simulink model "FYP"  (R2023b)
settings: Solver=FixedStepAuto  StartTime=0.0  StopTime=Inf  RelTol=1e-3  EnableMultiTasking=on
libraries: canmsglib x26, raspberrypiCommlib x26
(part 1 of 4)
settings Model: SimulationMode=external  ExtModeTrigDuration=2  Creator=aaron  LastModifiedBy=aaron
settings SolverCC: PositivePriorityOrder=on
settings OptimizationCC: EnhancedBackFolding=on  PassReuseOutputArgsAs=Individual arguments  ZeroExternalMemoryAtStartup=off  ZeroInternalMemoryAtStartup=off  MaxStackSize=64  OptimizeBlockOrder=speed  DifferentSizesBufferReuse=on  OptimizationCustomize=off  EfficientTunableParamExpr=on
settings DebuggingCC: UnderspecifiedInitializationDetection=Classic  MergeDetectMultiDrivingBlocksExec=none  ParameterTunabilityLossMsg=error
settings HardwareCC: ProdBitPerPointer=32  ProdBitPerSizeT=32  ProdBitPerPtrDiffT=32  ProdLargestAtomicInteger=Long  ProdLargestAtomicFloat=Double  ProdWordSize=32  ProdLongLongMode=on  ProdHWDeviceType=ARM Compatible->ARM Cortex
settings ModelReferenceCC: PropagateSignalLabelsOutOfModel=off
settings RTWCC: Description=Embedded Coder  SystemTargetFile=ert.tlc  HardwareBoard=Raspberry Pi  TemplateMakefile=ert_default_tmf  Toolchain=GNU GCC Embedded Linux  BuildConfiguration=Faster Runs
settings CodeAppCC: ForceParamTrailComments=on  IgnoreCustomStorageClasses=off  OperatorAnnotations=on  SimulinkDataObjDesc=on  SFDataObjDesc=on  InsertBlockDesc=on
settings ERTTargetCC: SupportContinuousTime=on  SupportVariableSizeSignals=on  ExtMode=on  ExtModeTransport=2  ExtModeStaticAlloc=on  ExtModeMaxTrigDuration=1000  ExtModeMexFile=ext_xcp  ExtModeMexArgs='192.168.167.94' 0 17725  ExtModeIntrfLevel=Level2 - Open

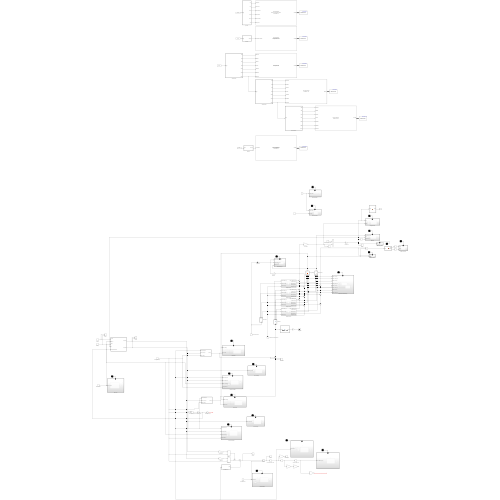
[thumbnail: Simulink's stored preview of the top-level diagram]
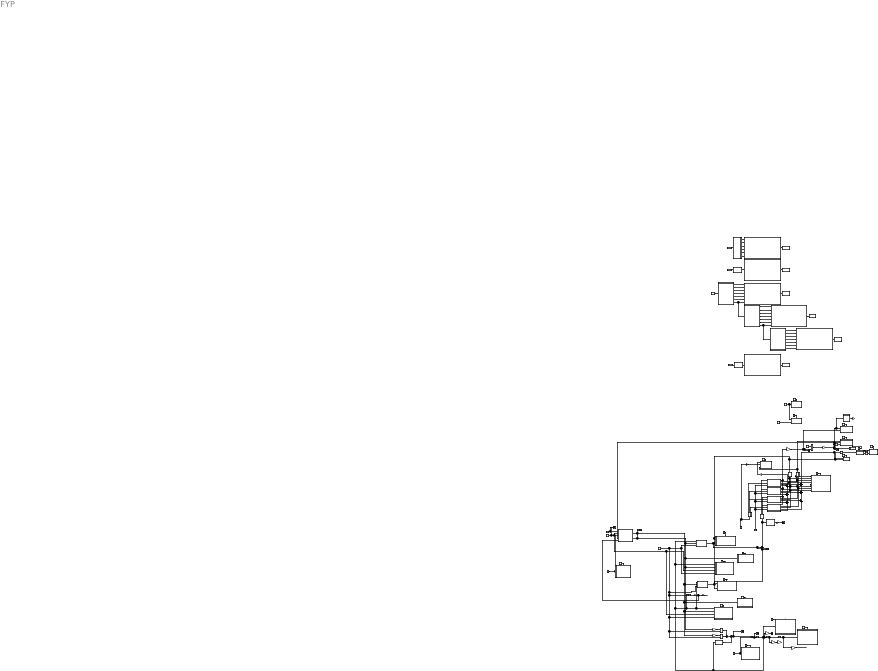
== system FYP ==
  A=F/m : Product  Inputs=*/
  Abs : Abs  SaturateOnIntegerOverflow=off
  Accel (m/s^2)to Vel (m/s) : Integrator
  Average Temp : MATLAB Function  TreatAsAtomicUnit=on
  Average Voltage : MATLAB Function  TreatAsAtomicUnit=on
  B SOC : Scope
  BMS Contactors 1 : Subsystem  TreatAsAtomicUnit=on
  BMS Contactors 2 : Subsystem  TreatAsAtomicUnit=on
  BMS Cooling Sys : Subsystem  TreatAsAtomicUnit=on
  BMS Energy Status : Subsystem  TreatAsAtomicUnit=on
  BMS Module State Monitoring : Subsystem  TreatAsAtomicUnit=on
  BMS SOC : Subsystem  TreatAsAtomicUnit=on
  BMS Sum Charge : Subsystem  TreatAsAtomicUnit=on
  BMS Sys Limits 2 : Subsystem  TreatAsAtomicUnit=on
  Battery Module 1 : Subsystem
  Battery Module 2 : Subsystem
  Battery Module 3 : Subsystem
  Battery Module 4 : Subsystem
  Brake () : Constant  Value=0
  CAN Pack1 : canmsglib/CAN Pack  MsgList=(none)  MsgName=ID405VIN  MsgIDType=Standard (11-bit identifier)  MsgIdentifier=1029  MsgLength=8  Remote=off  ApplyMinMax=off  BusOutput=on  SignalInfo={ 'VINA1405', '8', '32', 'LE', 'unsigned', 'Multiplexed', '16', '1', '0', '0', '4.29497E+009'; 'VINB405', '8', '32', 'LE', 'unsigned', 'Multiplexed', '17', '1', '0', '0', '4.29497E+009'; 'VINC405', '8', '32', 'LE', 'unsigned', 'Multiplexed', '18', '1', '0', '0', '4.29497E+009'; 'mux405', '0', '8', 'LE', 'unsigned', 'Multiplexor', '0', '1', '0', '0', '255'; 'VINA2405', '40', '24', 'LE', 'unsigned', 'Multiplexed', '16', '1', '0', '0', '1.67772E+007'; 'VINB2405', '40', '24', 'LE', 'unsigned', 'Multiplexed', '17', '1', '0', '-0', '1.67772E+007'; 'VINC2405', '40', '24', 'LE', 'unsigned', 'Multiplexed', '18', '1', '0', '0', '1.67772E+007' }
      settings: LibrarySourceBlock=canlib/CAN Pack  DataFormat=manually specified signals
  CAN Pack107 : canmsglib/CAN Pack  CANdbFile=C:\Users\aaron\OneDrive - Loughborough University\Work\Part D\FYP\tesla sniffing\Model3CAN.dbc  MsgList=ID3D8Elevation  MsgName=ID3D8Elevation  MsgIDType=Standard (11-bit identifier)  MsgIdentifier=984  MsgLength=2  Remote=off  ApplyMinMax=off  BusOutput=on  SignalInfo={'Elevation3D8','0','14','LE','signed','Standard','0','1','0','-8192','8191'}
      settings: LibrarySourceBlock=canlib/CAN Pack  DataFormat=CANdb specified signals
  CAN Pack115 : canmsglib/CAN Pack  MsgList=(none)  MsgName=ID405VIN  MsgIDType=Standard (11-bit identifier)  MsgIdentifier=1029  MsgLength=8  Remote=off  ApplyMinMax=off  BusOutput=on  SignalInfo={ 'VINA1405', '8', '32', 'LE', 'unsigned', 'Multiplexed', '16', '1', '0', '0', '4.29497E+009'; 'VINB405', '8', '32', 'LE', 'unsigned', 'Multiplexed', '17', '1', '0', '0', '4.29497E+009'; 'VINC405', '8', '32', 'LE', 'unsigned', 'Multiplexed', '18', '1', '0', '0', '4.29497E+009'; 'mux405', '0', '8', 'LE', 'unsigned', 'Multiplexor', '0', '1', '0', '0', '255'; 'VINA2405', '40', '24', 'LE', 'unsigned', 'Multiplexed', '16', '1', '0', '0', '1.67772E+007'; 'VINB2405', '40', '24', 'LE', 'unsigned', 'Multiplexed', '17', '1', '0', '-0', '1.67772E+007'; 'VINC2405', '40', '24', 'LE', 'unsigned', 'Multiplexed', '18', '1', '0', '0', '1.67772E+007' }
      settings: LibrarySourceBlock=canlib/CAN Pack  DataFormat=manually specified signals
  CAN Pack119 : canmsglib/CAN Pack  CANdbFile=C:\Users\aaron\OneDrive - Loughborough University\Work\Part D\FYP\tesla sniffing\Model3CAN.dbc  MsgList=ID528UnixTime  MsgName=ID528UnixTime  MsgIDType=Standard (11-bit identifier)  MsgIdentifier=1320  MsgLength=4  Remote=off  ApplyMinMax=off  BusOutput=on  SignalInfo={'UnixTimeSeconds528','24','32','BE','unsigned','Standard','0','1','0','0','4294970000'}
      settings: LibrarySourceBlock=canlib/CAN Pack  DataFormat=CANdb specified signals
  CAN Pack2 : canmsglib/CAN Pack  MsgList=(none)  MsgName=ID405VIN  MsgIDType=Standard (11-bit identifier)  MsgIdentifier=1029  MsgLength=8  Remote=off  ApplyMinMax=off  BusOutput=on  SignalInfo={ 'VINA1405', '8', '32', 'LE', 'unsigned', 'Multiplexed', '16', '1', '0', '0', '4.29497E+009'; 'VINB405', '8', '32', 'LE', 'unsigned', 'Multiplexed', '17', '1', '0', '0', '4.29497E+009'; 'VINC405', '8', '32', 'LE', 'unsigned', 'Multiplexed', '18', '1', '0', '0', '4.29497E+009'; 'mux405', '0', '8', 'LE', 'unsigned', 'Multiplexor', '0', '1', '0', '0', '255'; 'VINA2405', '40', '24', 'LE', 'unsigned', 'Multiplexed', '16', '1', '0', '0', '1.67772E+007'; 'VINB2405', '40', '24', 'LE', 'unsigned', 'Multiplexed', '17', '1', '0', '-0', '1.67772E+007'; 'VINC2405', '40', '24', 'LE', 'unsigned', 'Multiplexed', '18', '1', '0', '0', '1.67772E+007' }
      settings: LibrarySourceBlock=canlib/CAN Pack  DataFormat=manually specified signals
  CAN Pack82 : canmsglib/CAN Pack  CANdbFile=C:\Users\aaron\OneDrive - Loughborough University\Work\Part D\FYP\tesla sniffing\Model3CAN.dbc  MsgList=ID318SystemTimeUTC  MsgName=ID318SystemTimeUTC  MsgIDType=Standard (11-bit identifier)  MsgIdentifier=792  MsgLength=8  Remote=off  ApplyMinMax=off  BusOutput=on  SignalInfo={'UTCday318','32','8','LE','unsigned','Standard','0','1','0','-Inf','Inf';'UTChour318','24','8','LE','unsigned','Standard','0','1','0','-Inf','Inf';'UTCminutes318','40','8','LE','unsigned','Standard','0','1','0','-Inf','Inf';'UTCmonth318','8','8','LE','unsigned','Standard','0','1','0','-Inf','Inf';'UTCseconds318','16','8','LE','unsigned','Standard','0','1','0','-Inf','Inf';'UTCyear318','0','8','LE','unsigned','Standard','0','1','0','-Inf','Inf'}
      settings: LibrarySourceBlock=canlib/CAN Pack  DataFormat=CANdb specified signals
  CAN Transmit{1..2,82,107,115,119} (6 alike) : raspberrypiCommlib/CAN Transmit  DeviceID=can0  SetupCAN=off  TypeofCAN=Real  InputDataType=CAN Msg  BlockingMode_=off  BlockTimeout_=1  OutputStatus=off  IdentifierType=Standard (11-bit identifier)  MessageId=100  MsgLength=8  RemoteFrame=off  SimulateUsing=Code generation
  Coastdown Func : MATLAB Function  TreatAsAtomicUnit=on
  Constant : Constant
  Constant1 : Constant  Value=0
  Coolant Dist : MATLAB Function  TreatAsAtomicUnit=on
  Decimal to % : Gain  Gain=100
  Digital Clock1 : DigitalClock  SampleTime=1.02
  Digital Clock2 : DigitalClock
  Digital Clock3 : DigitalClock  SampleTime=1.01
  Digital Clock4 : DigitalClock
  Divide : Product  Inputs=/*
  Elevation : MATLAB Function  TreatAsAtomicUnit=on
  F=M/D front : Product  Inputs=*/
  F=M/D rear : Product  Inputs=*/
  Front PT Elec : Subsystem  TreatAsAtomicUnit=on
  Front PT Kinematics : Subsystem  TreatAsAtomicUnit=on
  Front PT Torque : Subsystem  TreatAsAtomicUnit=on
  Gain2 : Gain
  Gain3 : Gain  Gain=1/1000
  Gain5 : Gain  Gain=3.6
  Gain6 : Gain
  Gain7 : Gain  Gain=3.6
  Gain8 : Gain  Gain=3.6
  Gear Lever : Subsystem
  Gear Lever Pos : Constant  Value=3
  Integrator : Integrator
  Integrator1 : Integrator
  Integrator2 : Integrator
  M Pwr Draw : Scope  NumInputPorts=2
  MATLAB Function : MATLAB Function  TreatAsAtomicUnit=on
  MATLAB Function1 : MATLAB Function  TreatAsAtomicUnit=on
  MATLAB Function2 : MATLAB Function  TreatAsAtomicUnit=on
  MATLAB Function3 : MATLAB Function  TreatAsAtomicUnit=on
  MATLAB Function4 : MATLAB Function  TreatAsAtomicUnit=on
  MATLAB Function5 : MATLAB Function  TreatAsAtomicUnit=on
  Max Battery Capac (kWh) : Constant  Value=88
  Motor Speed (rpm) : Gain  Gain=9.54
  Motor speed (rad/s) : Gain  Gain=9.03
  Power Distr : MATLAB Function  TreatAsAtomicUnit=on
  Product : Product
  Pulse Generator{,1..18} (19 alike) : DiscretePulseGenerator  PulseType=Time based  Period=1
  Range Estimations : Subsystem  TreatAsAtomicUnit=on
  Rear PT Elec : Subsystem  TreatAsAtomicUnit=on
  Rear PT Kinematics : Subsystem  TreatAsAtomicUnit=on
  Rear PT Torque : Subsystem  TreatAsAtomicUnit=on
  Rolling Radius (m) : Constant  Value=0.3366
  Scope : Scope
  Subsystem : Subsystem
  Subsystem1 : Subsystem
  Sum{,1..9,11} (11 alike) : Sum  Inputs=++|
  Sum10 : Sum  Inputs=|+-
  Sys Time : MATLAB Function  TreatAsAtomicUnit=on
  Throttle () : Constant  Value=0
  Unix Time : MATLAB Function  TreatAsAtomicUnit=on
  V Accel : Scope
  V Force : Scope
  VIN Generation : MATLAB Function  TreatAsAtomicUnit=on
  VIN Generation1 : MATLAB Function  TreatAsAtomicUnit=on
  VIN Generation2 : MATLAB Function  TreatAsAtomicUnit=on
  Vehicle Estimates : Subsystem  TreatAsAtomicUnit=on
  Vehicle Mass )kg) : Constant  Value=1851+80*4
  Vehicle Speed : Scope
  Vel (m/s) to Disp (m) : Integrator
  W to kW : Gain  Gain=0.001
  Wh to kWh : Gain  Gain=1/1000
  assume constant flow : Constant  Value=50
  constant temp coolant from rad : Constant  Value=50
  energy perc : Scope
  gear ratio : Gain  Gain=9.03
  gear ratio1 : Gain  Gain=9.03
  kg/s to l/min : Gain  Gain=60
  pedals : Scope  NumInputPorts=2
  torques : Scope  NumInputPorts=2
  untitledPanel : Subsystem  Tag=HiddenForWebPanel  IsWebBlockPanel=on
  wheel speed (rad/s) : Product  Inputs=*/
  wires:
  Pulse Generator13/1 -> BMS Cooling Sys/Trigger
  Sum3/1 -> Wh to kWh/1
  Power Distr/2(p2) -> Battery Module 2/1(Power Request (W))
  Pulse Generator5/1 -> Front PT Kinematics/Trigger
  Sum1/1 -> Sum/2
  Pulse Generator1/1 -> Rear PT Torque/Trigger
  Pulse Generator/1 -> Rear PT Elec/Trigger
  Pulse Generator2/1 -> Rear PT Kinematics/Trigger
  Rolling Radius (m)/1 -> Rear PT Kinematics/4(Rolling Radius (m)), MATLAB Function5/3(rolling_radius_m), MATLAB Function4/3(rolling_radius_m), wheel speed (rad/s)/2, Front PT Kinematics/4(Rolling Radius (m)), F=M/D rear/2, F=M/D front/2
  Integrator/1 -> BMS SOC/3(Integrated SOC)
  Battery Module 2/4(Module Current (A)) -> Sum1/1
  Divide/1 -> Decimal to %/1
  Pulse Generator6/1 -> BMS Module State Monitoring/Trigger
  CAN Pack119/1 -> CAN Transmit119/1
  VIN Generation/1(VINA) -> CAN Pack115/1
  Sum2/1 -> Sum1/2
  Battery Module 4/3(Module Voltage (V)) -> BMS Module State Monitoring/8(Module 4 Voltage (V)), Average Voltage/4(v4)
  Battery Module 2/5(Heating Power (W)) -> Sum7/1
  Brake ()/1 -> pedals/2, Front PT Kinematics/3(Brake Pedal Pos (%)), Rear PT Kinematics/3(Brake Pedal Pos (%)), MATLAB Function1/2(brakePct)
  Product/1 -> MATLAB Function/1(power)
  MATLAB Function1/2(torqueRear) -> torques/2, Rear PT Torque/1(Motor Torque (Nm)), gear ratio1/1, Rear PT Kinematics/2(Motor Torque (m/s)), MATLAB Function5/2(motor_torque_Nm)
  Sum7/1 -> Sum8/2
  Battery Module 2/2(Module Temp (C)) -> Average Temp/2(v2), BMS Module State Monitoring/3(Module 2 Temp (C))
  MATLAB Function/1(charge) -> Integrator1/1
  CAN Pack107/1 -> CAN Transmit107/1
  Coolant Dist/3(p3) -> Battery Module 3/2(Coolant Flow (kg/s))
  Pulse Generator7/1 -> BMS Sys Limits 2/Trigger
  Integrator1/1 -> BMS Sum Charge/1(Power1)
  Integrator2/1 -> BMS Sum Charge/2(Power2)
  Pulse Generator9/1 -> BMS Energy Status/Trigger
  W to kW/1 -> BMS Cooling Sys/1(Battery Heating Power (kW))
  kg/s to l/min/1 -> BMS Cooling Sys/2(Coolant Vol Flow (LPM))
  Battery Module 3/1(Energy Remaining (Wh)) -> Sum5/1
  Battery Module 3/4(Module Current (A)) -> Sum2/1
  Pulse Generator11/1 -> BMS Contactors 2/Trigger
  Coolant Dist/2(p2) -> Battery Module 2/2(Coolant Flow (kg/s))
  Pulse Generator12/1 -> BMS Contactors 1/Trigger
  Sum6/1 -> Sum7/2
  Battery Module 4/5(Heating Power (W)) -> Sum6/2
  Battery Module 1/3(Module Voltage (V)) -> BMS Module State Monitoring/2(Module 1 Voltage (V)), Average Voltage/1(v1)
  Battery Module 3/5(Heating Power (W)) -> Sum6/1
  MATLAB Function4/1(power_W) -> Front PT Elec/2(Motor Power), M Pwr Draw/2, Sum9/2
  MATLAB Function1/1(torqueFront) -> torques/1, MATLAB Function4/2(motor_torque_Nm), Front PT Torque/1(Motor Torque (Nm)), gear ratio/1, Front PT Kinematics/2(Motor Torque (m/s))
  Max Battery Capac (kWh)/1 -> Divide/1
  Constant/1 -> BMS Contactors 2/1(Contactor State), BMS Contactors 1/1(Contactor State)
  Wh to kWh/1 -> Range Estimations/2(Energy), Scope/1, Divide/2
  CAN Pack115/1 -> CAN Transmit115/1
  Coolant Dist/1(p1) -> Battery Module 1/2(Coolant Flow (kg/s))
  Power Distr/3(p3) -> Battery Module 3/1(Power Request (W))
  Coolant Dist/4(p4) -> Battery Module 4/2(Coolant Flow (kg/s))
  Sys Time/6(year) -> CAN Pack82/6
  Battery Module 2/1(Energy Remaining (Wh)) -> Sum4/1
  Battery Module 2/3(Module Voltage (V)) -> BMS Module State Monitoring/4(Module 2 Voltage (V)), Average Voltage/2(v2)
  Average Temp/1(v) -> BMS SOC/1(Current Battery Temp), BMS Cooling Sys/3(Battery Temp (C))
  constant temp coolant from rad/1 -> Battery Module 1/3(Coolant Temp (C)), Battery Module 2/3(Coolant Temp (C)), Battery Module 3/3(Coolant Temp (C)), Battery Module 4/3(Coolant Temp (C))
  Power Distr/1(p1) -> Battery Module 1/1(Power Request (W))
  Elevation/1(Elevation) -> CAN Pack107/1
  Battery Module 4/4(Module Current (A)) -> Sum2/2
  Battery Module 3/3(Module Voltage (V)) -> BMS Module State Monitoring/6(Module 3 Voltage (V)), Average Voltage/3(v3)
  MATLAB Function/2(discharge) -> Integrator2/1
  Battery Module 3/2(Module Temp (C)) -> Average Temp/3(v3), BMS Module State Monitoring/5(Module 3 Temp (C))
  Battery Module 1/4(Module Current (A)) -> Sum/1
  Pulse Generator8/1 -> BMS Sum Charge/Trigger
  Pulse Generator3/1 -> Front PT Elec/Trigger
  MATLAB Function5/1(power_W) -> M Pwr Draw/1, Sum9/1, Rear PT Elec/2(Motor Power)
  Digital Clock3/1 -> Elevation/1(trigger)
  Accel (m/s^2)to Vel (m/s)/1 -> Coastdown Func/1(v), MATLAB Function5/1(vehicle_speed_mps), Rear PT Kinematics/1(Vehicle Speed (m/s)), wheel speed (rad/s)/1, MATLAB Function4/1(vehicle_speed_mps), Front PT Kinematics/1(Vehicle Speed (m/s)), Subsystem1/1(vehicle speed), Gain5/1, Abs/1
  Constant1/1 -> BMS Contactors 2/2(FC request)
  Battery Module 4/1(Energy Remaining (Wh)) -> Sum5/2
  Sum8/1 -> W to kW/1
  Sys Time/2(hour) -> CAN Pack82/2
  VIN Generation/2(VINB) -> CAN Pack115/2
  Battery Module 1/5(Heating Power (W)) -> Sum8/1
  Power Distr/4(p4) -> Battery Module 4/1(Power Request (W))
  CAN Pack82/1 -> CAN Transmit82/1
  Sys Time/3(minute) -> CAN Pack82/3
  Sum4/1 -> Sum3/2
  Digital Clock2/1 -> Sys Time/1(trigger)
  Sum5/1 -> Sum4/2
  Sum/1 -> BMS Sys Limits 2/1(Current), Product/1
  Unix Time/1(UnixTime) -> CAN Pack119/1
  Digital Clock1/1 -> Unix Time/1(trigger)
  Sys Time/1(day) -> CAN Pack82/1
  VIN Generation/3(VINC) -> CAN Pack115/3
  Average Voltage/1(v) -> Product/2, BMS Sys Limits 2/2(Voltage), Front PT Elec/1(Battery Voltage), Rear PT Elec/1(Battery Voltage)
  Digital Clock4/1 -> VIN Generation/1(trigger)
  Sys Time/5(second) -> CAN Pack82/5
  Pulse Generator4/1 -> Front PT Torque/Trigger
  Battery Module 1/1(Energy Remaining (Wh)) -> Sum3/1
  Sys Time/4(month) -> CAN Pack82/4
  Battery Module 4/2(Module Temp (C)) -> Average Temp/4(v4), BMS Module State Monitoring/7(Module 4 Temp (C))
  Pulse Generator10/1 -> BMS SOC/Trigger
  assume constant flow/1 -> Coolant Dist/1(pr), kg/s to l/min/1
  Battery Module 1/2(Module Temp (C)) -> BMS Module State Monitoring/1(Module 1 Temp (C)), Average Temp/1(v1)
  Throttle ()/1 -> pedals/1, MATLAB Function1/1(accelPct)
  A=F/m/1 -> V Accel/1, Accel (m/s^2)to Vel (m/s)/1
  Vehicle Mass )kg)/1 -> A=F/m/2, Vehicle Estimates/1(Vehicle Mass)
  Coastdown Func/1(F_total) -> Sum10/2
  Sum10/1 -> V Force/1, A=F/m/1
  gear ratio/1 -> F=M/D front/1
  F=M/D front/1 -> Sum11/2
  gear ratio1/1 -> F=M/D rear/1
  F=M/D rear/1 -> Sum11/1
  Pulse Generator14/1 -> Subsystem/Trigger
  Pulse Generator15/1 -> Vehicle Estimates/Trigger
  Pulse Generator16/1 -> Gear Lever/Trigger
  Gear Lever Pos/1 -> MATLAB Function1/3(PRND), Gear Lever/1(Gear Lever Pos)
  Pulse Generator17/1 -> Subsystem1/Trigger
  Pulse Generator18/1 -> Range Estimations/Trigger
  VIN Generation/7(VINC2) -> VIN Generation1/1(trigger), CAN Pack115/7
  VIN Generation/6(VINB2) -> CAN Pack115/6
  VIN Generation/5(VINA2) -> CAN Pack115/5
  VIN Generation/4(MUX) -> CAN Pack115/4
  VIN Generation1/4(MUX) -> CAN Pack1/4
  VIN Generation1/6(VINB2) -> CAN Pack1/6
  CAN Pack1/1 -> CAN Transmit1/1
  VIN Generation1/2(VINB) -> CAN Pack1/2
  VIN Generation1/5(VINA2) -> CAN Pack1/5
  VIN Generation1/1(VINA) -> CAN Pack1/1
  VIN Generation1/3(VINC) -> CAN Pack1/3
  VIN Generation1/7(VINC2) -> VIN Generation2/1(trigger), CAN Pack1/7
  VIN Generation2/5(VINA2) -> CAN Pack2/5
  VIN Generation2/4(MUX) -> CAN Pack2/4
  VIN Generation2/3(VINC) -> CAN Pack2/3
  VIN Generation2/6(VINB2) -> CAN Pack2/6
  VIN Generation2/2(VINB) -> CAN Pack2/2
  CAN Pack2/1 -> CAN Transmit2/1
  VIN Generation2/1(VINA) -> CAN Pack2/1
  VIN Generation2/7(VINC2) -> CAN Pack2/7
  MATLAB Function2/1(percent) -> Gain2/1
  Sum9/1 -> MATLAB Function2/1(currentW), Power Distr/1(pr)
  Vel (m/s) to Disp (m)/1 -> Gain3/1, Subsystem/1(vehicle displacement (m))
  Gain3/1 -> ?
  Gain5/1 -> Vehicle Speed/1
  Sum11/1 -> Sum10/1
  MATLAB Function3/1(Range) -> Gain6/1
  Abs/1 -> Gain7/1, Vel (m/s) to Disp (m)/1
  Gain7/1 -> Gain8/1
  wheel speed (rad/s)/1 -> Motor speed (rad/s)/1
  Decimal to %/1 -> BMS Energy Status/1(SOC), B SOC/1, Integrator/1, BMS SOC/2(SOC), MATLAB Function1/4(soc), MATLAB Function3/1(Energy), Range Estimations/1(SOC)
  Motor speed (rad/s)/1 -> MATLAB Function1/5(motorSpeedRadPerSec), Motor Speed (rpm)/1
  Motor Speed (rpm)/1 -> ?
  Gain2/1 -> energy perc/1

== system FYP/BMS Contactors 1 ==
  Contactor State : Inport
  Trigger : TriggerPort  VariantControl=(inherit)
  CAN Pack1 : canmsglib/CAN Pack  CANdbFile=C:\Users\aaron\OneDrive - Loughborough University\Work\Part D\FYP\tesla sniffing\Model3CAN.dbc  MsgList=ID016DI_bmsRequest  MsgName=ID016DI_bmsRequest  MsgIDType=Standard (11-bit identifier)  MsgIdentifier=22  MsgLength=1  Remote=off  ApplyMinMax=off  BusOutput=on  SignalInfo={'DI_bmsOpenContactorsRequest','4','1','LE','unsigned','Standard','0','1','0','0','1';'DI_bmsRequestInterfaceVersion','0','4','LE','unsigned','Standard','0','1','0','0','15'}
      settings: LibrarySourceBlock=canlib/CAN Pack  DataFormat=CANdb specified signals
  CAN Transmit1 : raspberrypiCommlib/CAN Transmit  DeviceID=can0  SetupCAN=off  TypeofCAN=Real  InputDataType=CAN Msg  BlockingMode_=off  BlockTimeout_=1  OutputStatus=off  IdentifierType=Standard (11-bit identifier)  MessageId=100  MsgLength=8  RemoteFrame=off  SimulateUsing=Code generation
  Version (Value needs tuning!) : Constant  Value=3
  wires:
  CAN Pack1/1 -> CAN Transmit1/1
  Contactor State/1 -> CAN Pack1/1
  Version (Value needs tuning!)/1 -> CAN Pack1/2

== system FYP/BMS Contactors 2 ==
  Contactor State : Inport
  FC request : Inport  Port=2
  Trigger : TriggerPort  VariantControl=(inherit)
  CAN Pack40 : canmsglib/CAN Pack  CANdbFile=C:\Users\aaron\OneDrive - Loughborough University\Work\Part D\FYP\tesla sniffing\Model3CAN.dbc  MsgList=ID232BMS_contactorRequest  MsgName=ID232BMS_contactorRequest  MsgIDType=Standard (11-bit identifier)  MsgIdentifier=562  MsgLength=8  Remote=off  ApplyMinMax=off  BusOutput=on  SignalInfo={'BMS_ensShouldBeActiveForDrive','7','1','LE','unsigned','Standard','0','1','0','0','1';'BMS_fcContactorRequest','0','3','LE','unsigned','Standard','0','1','0','0','5';'BMS_fcLinkOkToEnergizeRequest','32','2','LE','unsigned','Standard','0','1','0','0','2';'BMS_gpoHasCompleted','6','1','LE','unsigned','Standard','0','1','0','0','1';'BMS_internalHvilSenseV','16','16','LE','unsigned','Standard','0','0.001','0','0','65.534';'BMS_packContactorRequest','3','3','LE','unsigned','Standard','0','1','0','0','5';'BMS_pcsPwmDisable','8','1','LE','unsigned','Standard','0','1','0','0','1'}
      settings: LibrarySourceBlock=canlib/CAN Pack  DataFormat=CANdb specified signals
  CAN Transmit40 : raspberrypiCommlib/CAN Transmit  DeviceID=can0  SetupCAN=off  TypeofCAN=Real  InputDataType=CAN Msg  BlockingMode_=off  BlockTimeout_=1  OutputStatus=off  IdentifierType=Standard (11-bit identifier)  MessageId=100  MsgLength=8  RemoteFrame=off  SimulateUsing=Code generation
  wires:
  CAN Pack40/1 -> CAN Transmit40/1
  Contactor State/1 -> CAN Pack40/6
  FC request/1 -> CAN Pack40/3, CAN Pack40/2

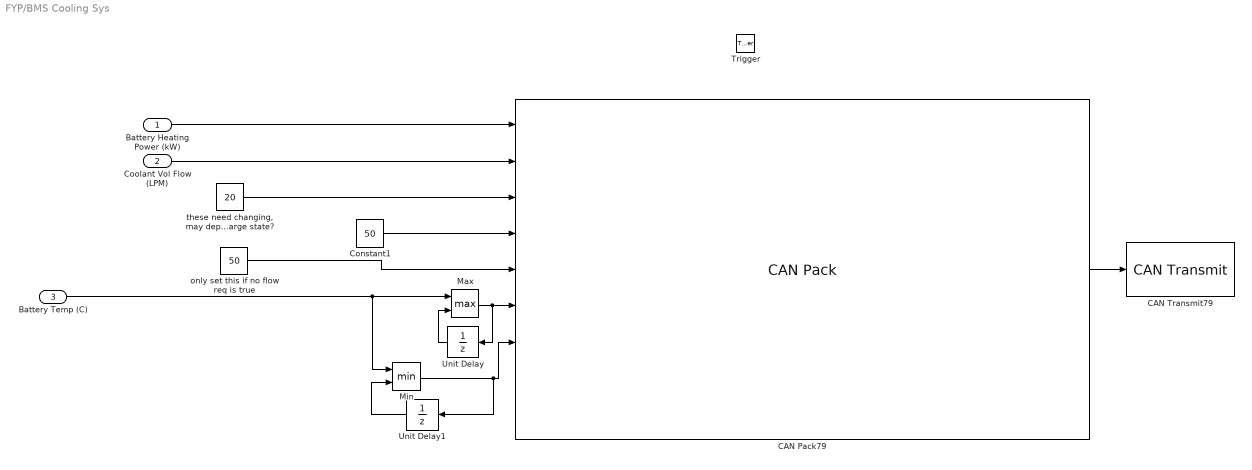
== system FYP/BMS Cooling Sys ==
  Battery Heating Power (kW) : Inport
  Coolant Vol Flow (LPM) : Inport  Port=2
  Battery Temp (C) : Inport  Port=3
  Trigger : TriggerPort  VariantControl=(inherit)
  CAN Pack79 : canmsglib/CAN Pack  CANdbFile=C:\Users\aaron\OneDrive - Loughborough University\Work\Part D\FYP\tesla sniffing\Model3CAN.dbc  MsgList=ID312BMSthermal  MsgName=ID312BMSthermal  MsgIDType=Standard (11-bit identifier)  MsgIdentifier=786  MsgLength=8  Remote=off  ApplyMinMax=off  BusOutput=on  SignalInfo={'BMSdissipation312','0','10','LE','unsigned','Standard','0','0.02','0','0','20';'BMSflowRequest312','10','7','LE','unsigned','Standard','0','0.3','0','0','30';'BMSinletActiveCoolTarget312','17','9','LE','unsigned','Standard','0','0.25','-25','-25','100';'BMSinletActiveHeatTarget312','35','9','LE','unsigned','Standard','0','0.25','-25','-25','100';'BMSinletPassiveTarget312','26','9','LE','unsigned','Standard','0','0.25','-25','-25','100';'BMSmaxPackTemperature','53','9','LE','unsigned','Standard','0','0.25','-25','-25','100';'BMSminPackTemperature','44','9','LE','unsigned','Standard','0','0.25','-25','-25','100';'BMSnoFlowRequest312','63','1','LE','unsigned','Standard','0','1','0','0','1';'BMSpcsNoFlowRequest312','62','1','LE','unsigned','Standard','0','1','0','0','1'}
      settings: LibrarySourceBlock=canlib/CAN Pack  DataFormat=CANdb specified signals
  CAN Transmit79 : raspberrypiCommlib/CAN Transmit  DeviceID=can0  SetupCAN=off  TypeofCAN=Real  InputDataType=CAN Msg  BlockingMode_=off  BlockTimeout_=1  OutputStatus=off  IdentifierType=Standard (11-bit identifier)  MessageId=100  MsgLength=8  RemoteFrame=off  SimulateUsing=Code generation
  Constant1 : Constant  Value=50
  Max : MinMax  Function=max  Inputs=2
  Min : MinMax  Inputs=2
  Unit Delay : UnitDelay  SampleTime=-1  HasFrameUpgradeWarning=on
  Unit Delay1 : UnitDelay  InitialCondition=90  SampleTime=-1  HasFrameUpgradeWarning=on
  only set this if no flow req is true : Constant  Value=50
  "these need changing, may depend on vehicle charge state?" : Constant  Value=20
  wires:
  CAN Pack79/1 -> CAN Transmit79/1
  Battery Heating Power (kW)/1 -> CAN Pack79/1
  Coolant Vol Flow (LPM)/1 -> CAN Pack79/2
  "these need changing, may depend on vehicle charge state?"/1 -> CAN Pack79/3
  Constant1/1 -> CAN Pack79/4
  Max/1 -> Unit Delay/1, CAN Pack79/6
  Battery Temp (C)/1 -> Max/1, Min/1
  Min/1 -> CAN Pack79/7, Unit Delay1/1
  only set this if no flow req is true/1 -> CAN Pack79/5
  Unit Delay/1 -> Max/2
  Unit Delay1/1 -> Min/2

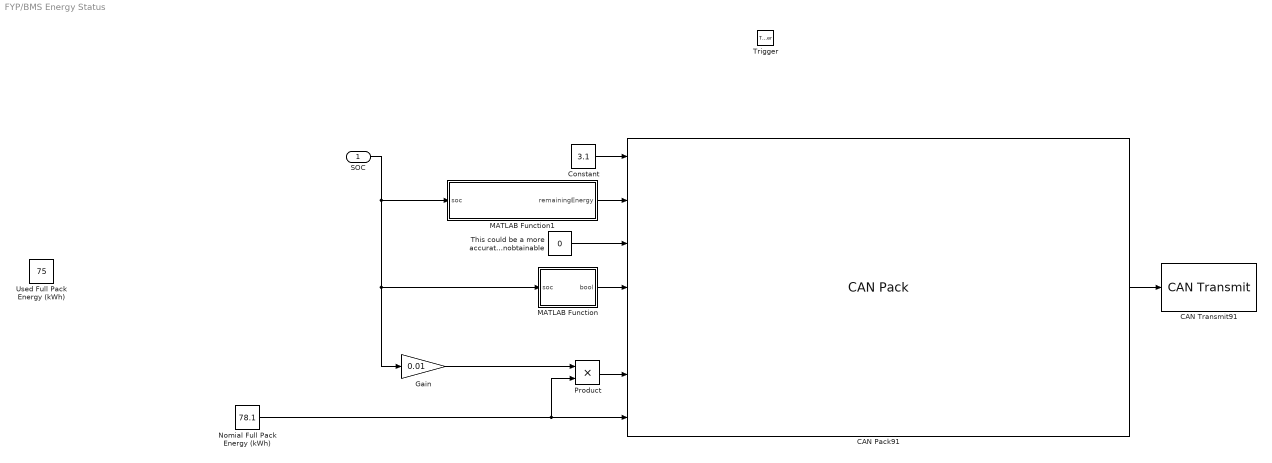
== system FYP/BMS Energy Status ==
  SOC : Inport
  Trigger : TriggerPort  VariantControl=(inherit)
  CAN Pack91 : canmsglib/CAN Pack  CANdbFile=C:\Users\aaron\OneDrive - Loughborough University\Work\Part D\FYP\tesla sniffing\Model3CAN.dbc  MsgList=ID352BMS_energyStatus  MsgName=ID352BMS_energyStatus  MsgIDType=Standard (11-bit identifier)  MsgIdentifier=850  MsgLength=8  Remote=off  ApplyMinMax=off  BusOutput=on  SignalInfo={'BMS_energyBuffer','55','8','LE','unsigned','Standard','0','0.1','0','0','25.4';'BMS_energyToChargeComplete','44','11','LE','unsigned','Standard','0','0.1','0','0','204.6';'BMS_expectedEnergyRemaining','22','11','LE','unsigned','Standard','0','0.1','0','0','204.6';'BMS_fullChargeComplete','63','1','LE','unsigned','Standard','0','1','0','0','1';'BMS_idealEnergyRemaining','33','11','LE','unsigned','Standard','0','0.1','0','0','204.6';'BMS_nominalEnergyRemaining','11','11','LE','unsigned','Standard','0','0.1','0','0','204.6';'BMS_nominalFullPackEnergy','0','11','LE','unsigned','Standard','0','0.1','0','0','204.6'}
      settings: LibrarySourceBlock=canlib/CAN Pack  DataFormat=CANdb specified signals
  CAN Transmit91 : raspberrypiCommlib/CAN Transmit  DeviceID=can0  SetupCAN=off  TypeofCAN=Real  InputDataType=CAN Msg  BlockingMode_=off  BlockTimeout_=1  OutputStatus=off  IdentifierType=Standard (11-bit identifier)  MessageId=100  MsgLength=8  RemoteFrame=off  SimulateUsing=Code generation
  Constant : Constant  Value=3.1
  Gain : Gain  Gain=0.01
  MATLAB Function : MATLAB Function  TreatAsAtomicUnit=on
  MATLAB Function1 : MATLAB Function  TreatAsAtomicUnit=on
  Nomial Full Pack Energy (kWh) : Constant  Value=78.1
  Product : Product
  "This could be a more accurate value, no trip planning within model, so data unobtainable" : Constant  Value=0
  Used Full Pack Energy (kWh) : Constant  Value=75
  wires:
  CAN Pack91/1 -> CAN Transmit91/1
  Nomial Full Pack Energy (kWh)/1 -> Product/2, CAN Pack91/7
  Product/1 -> CAN Pack91/6
  Gain/1 -> Product/1
  SOC/1 -> MATLAB Function1/1(soc), MATLAB Function/1(soc), Gain/1
  MATLAB Function/1(bool) -> CAN Pack91/4
  MATLAB Function1/1(remainingEnergy) -> CAN Pack91/2
  Constant/1 -> CAN Pack91/1
  "This could be a more accurate value, no trip planning within model, so data unobtainable"/1 -> CAN Pack91/3

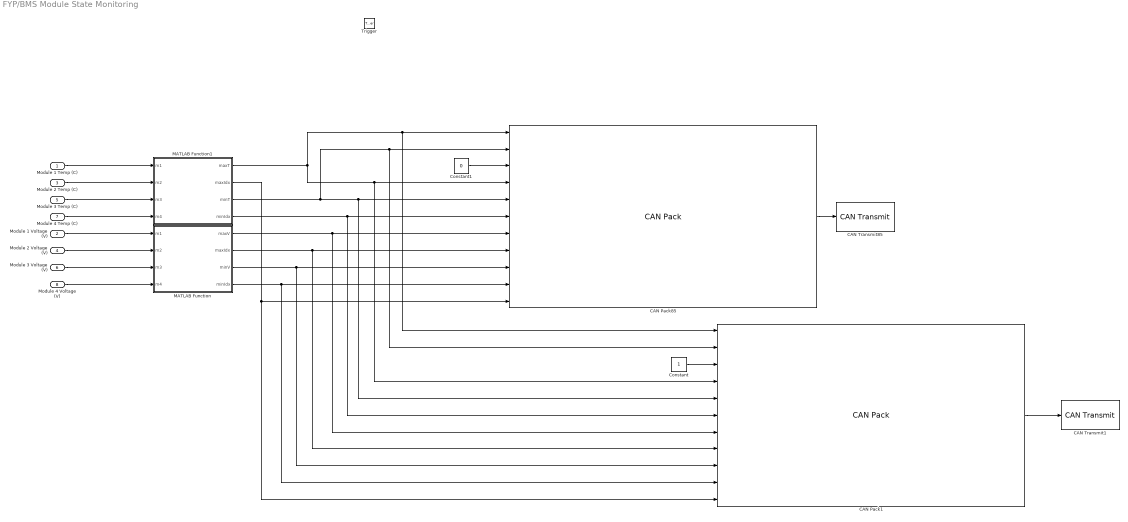
== system FYP/BMS Module State Monitoring ==
  Module 1 Temp (C) : Inport
  Module 1 Voltage (V) : Inport  Port=2
  Module 2 Temp (C) : Inport  Port=3
  Module 2 Voltage (V) : Inport  Port=4
  Module 3 Temp (C) : Inport  Port=5
  Module 3 Voltage (V) : Inport  Port=6
  Module 4 Temp (C) : Inport  Port=7
  Module 4 Voltage (V) : Inport  Port=8
  Trigger : TriggerPort  VariantControl=(inherit)
  CAN Pack1 : canmsglib/CAN Pack  CANdbFile=C:\Users\aaron\OneDrive - Loughborough University\Work\Part D\FYP\tesla sniffing\Model3CAN.dbc  MsgList=ID332BattBrickMinMax  MsgName=ID332BattBrickMinMax  MsgIDType=Standard (11-bit identifier)  MsgIdentifier=818  MsgLength=6  Remote=off  ApplyMinMax=off  BusOutput=on  SignalInfo={'BattBrickModelTMax332','32','8','LE','unsigned','Multiplexed','0','0.5','-40','-Inf','Inf';'BattBrickModelTMin332','40','8','LE','unsigned','Multiplexed','0','0.5','-40','-Inf','Inf';'BattBrickMultiplexer332','0','2','LE','unsigned','Multiplexor','0','1','0','-Inf','Inf';'BattBrickTempMax332','16','8','LE','unsigned','Multiplexed','0','0.5','-40','-Inf','Inf';'BattBrickTempMin332','24','8','LE','unsigned','Multiplexed','0','0.5','-40','-Inf','Inf';'BattBrickTempMinNum332','8','4','LE','unsigned','Multiplexed','0','1','0','-Inf','Inf';'BattBrickVoltageMax332','2','12','LE','unsigned','Multiplexed','1','0.002','0','-Inf','Inf';'BattBrickVoltageMaxNum332','32','7','LE','unsigned','Multiplexed','1','1','1','-Inf','Inf';'BattBrickVoltageMin332','16','12','LE','unsigned','Multiplexed','1','0.002','0','-Inf','Inf';'BattBrickVoltageMinNum332','40','7','LE','unsigned','Multiplexed','1','1','1','-Inf','Inf';'BattBrickempMaxNum332','2','4','LE','unsigned','Multiplexed','0','1','0','-Inf','Inf'}
      settings: LibrarySourceBlock=canlib/CAN Pack  DataFormat=CANdb specified signals
  CAN Pack85 : canmsglib/CAN Pack  CANdbFile=C:\Users\aaron\OneDrive - Loughborough University\Work\Part D\FYP\tesla sniffing\Model3CAN.dbc  MsgList=ID332BattBrickMinMax  MsgName=ID332BattBrickMinMax  MsgIDType=Standard (11-bit identifier)  MsgIdentifier=818  MsgLength=6  Remote=off  ApplyMinMax=off  BusOutput=on  SignalInfo={'BattBrickModelTMax332','32','8','LE','unsigned','Multiplexed','0','0.5','-40','-Inf','Inf';'BattBrickModelTMin332','40','8','LE','unsigned','Multiplexed','0','0.5','-40','-Inf','Inf';'BattBrickMultiplexer332','0','2','LE','unsigned','Multiplexor','0','1','0','-Inf','Inf';'BattBrickTempMax332','16','8','LE','unsigned','Multiplexed','0','0.5','-40','-Inf','Inf';'BattBrickTempMin332','24','8','LE','unsigned','Multiplexed','0','0.5','-40','-Inf','Inf';'BattBrickTempMinNum332','8','4','LE','unsigned','Multiplexed','0','1','0','-Inf','Inf';'BattBrickVoltageMax332','2','12','LE','unsigned','Multiplexed','1','0.002','0','-Inf','Inf';'BattBrickVoltageMaxNum332','32','7','LE','unsigned','Multiplexed','1','1','1','-Inf','Inf';'BattBrickVoltageMin332','16','12','LE','unsigned','Multiplexed','1','0.002','0','-Inf','Inf';'BattBrickVoltageMinNum332','40','7','LE','unsigned','Multiplexed','1','1','1','-Inf','Inf';'BattBrickempMaxNum332','2','4','LE','unsigned','Multiplexed','0','1','0','-Inf','Inf'}
      settings: LibrarySourceBlock=canlib/CAN Pack  DataFormat=CANdb specified signals
  CAN Transmit1 : raspberrypiCommlib/CAN Transmit  DeviceID=can0  SetupCAN=off  TypeofCAN=Real  InputDataType=CAN Msg  BlockingMode_=off  BlockTimeout_=1  OutputStatus=off  IdentifierType=Standard (11-bit identifier)  MessageId=100  MsgLength=8  RemoteFrame=off  SimulateUsing=Code generation
  CAN Transmit85 : raspberrypiCommlib/CAN Transmit  DeviceID=can0  SetupCAN=off  TypeofCAN=Real  InputDataType=CAN Msg  BlockingMode_=off  BlockTimeout_=1  OutputStatus=off  IdentifierType=Standard (11-bit identifier)  MessageId=100  MsgLength=8  RemoteFrame=off  SimulateUsing=Code generation
  Constant : Constant
  Constant1 : Constant  Value=0
  MATLAB Function : MATLAB Function  TreatAsAtomicUnit=on
  MATLAB Function1 : MATLAB Function  TreatAsAtomicUnit=on
  wires:
  CAN Pack85/1 -> CAN Transmit85/1
  CAN Pack1/1 -> CAN Transmit1/1
  Constant/1 -> CAN Pack1/3
  Constant1/1 -> CAN Pack85/3
  Module 1 Voltage (V)/1 -> MATLAB Function/1(m1)
  Module 2 Voltage (V)/1 -> MATLAB Function/2(m2)
  Module 3 Voltage (V)/1 -> MATLAB Function/3(m3)
  Module 4 Voltage (V)/1 -> MATLAB Function/4(m4)
  MATLAB Function/1(maxV) -> CAN Pack1/7, CAN Pack85/7
  MATLAB Function/2(maxIdx) -> CAN Pack85/8, CAN Pack1/8
  MATLAB Function/3(minV) -> CAN Pack1/9, CAN Pack85/9
  MATLAB Function/4(minIdx) -> CAN Pack1/10, CAN Pack85/10
  Module 4 Temp (C)/1 -> MATLAB Function1/4(m4)
  Module 3 Temp (C)/1 -> MATLAB Function1/3(m3)
  Module 2 Temp (C)/1 -> MATLAB Function1/2(m2)
  Module 1 Temp (C)/1 -> MATLAB Function1/1(m1)
  MATLAB Function1/1(maxT) -> CAN Pack1/4, CAN Pack85/4, CAN Pack85/1, CAN Pack1/1
  MATLAB Function1/3(minT) -> CAN Pack85/2, CAN Pack1/2, CAN Pack1/5, CAN Pack85/5
  MATLAB Function1/4(minIdx) -> CAN Pack1/6, CAN Pack85/6
  MATLAB Function1/2(maxIdx) -> CAN Pack1/11, CAN Pack85/11

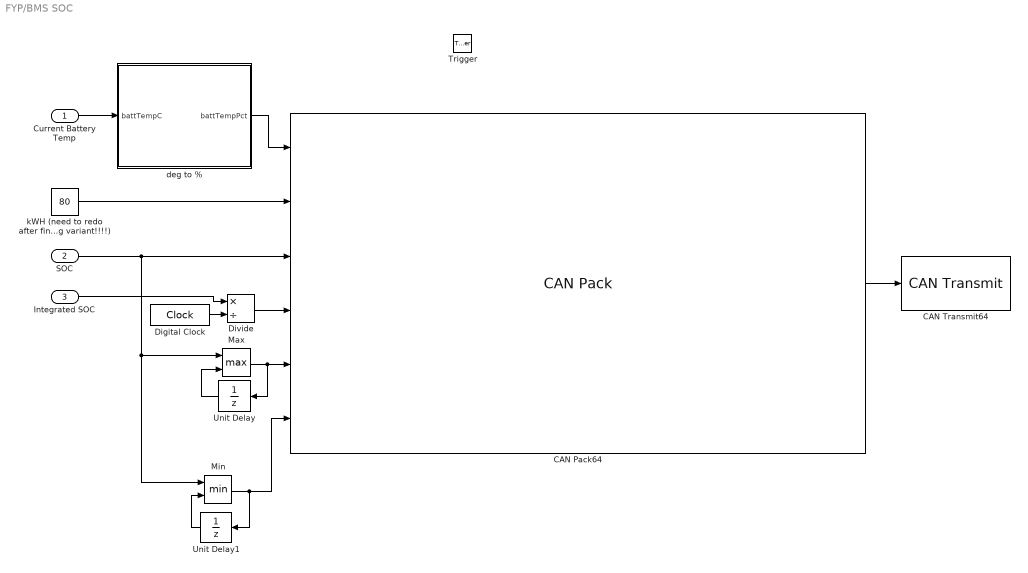
== system FYP/BMS SOC ==
  Current Battery Temp : Inport
  SOC : Inport  Port=2
  Integrated SOC : Inport  Port=3
  Trigger : TriggerPort  VariantControl=(inherit)
  CAN Pack64 : canmsglib/CAN Pack  CANdbFile=C:\Users\aaron\OneDrive - Loughborough University\Work\Part D\FYP\tesla sniffing\Model3CAN.dbc  MsgList=ID292BMS_SOC  MsgName=ID292BMS_SOC  MsgIDType=Standard (11-bit identifier)  MsgIdentifier=658  MsgLength=8  Remote=off  ApplyMinMax=off  BusOutput=on  SignalInfo={'BMS_battTempPct','50','8','LE','unsigned','Standard','0','0.4','0','0','100';'BattBeginningOfLifeEnergy292','40','10','LE','unsigned','Standard','0','0.1','0','0','102.3';'SOCUI292','10','10','LE','unsigned','Standard','0','0.1','0','0','102.3';'SOCave292','30','10','LE','unsigned','Standard','0','0.1','0','0','102.3';'SOCmax292','20','10','LE','unsigned','Standard','0','0.1','0','0','102.3';'SOCmin292','0','10','LE','unsigned','Standard','0','0.1','0','0','102.3'}
      settings: LibrarySourceBlock=canlib/CAN Pack  DataFormat=CANdb specified signals
  CAN Transmit64 : raspberrypiCommlib/CAN Transmit  DeviceID=can0  SetupCAN=off  TypeofCAN=Real  InputDataType=CAN Msg  BlockingMode_=off  BlockTimeout_=1  OutputStatus=off  IdentifierType=Standard (11-bit identifier)  MessageId=100  MsgLength=8  RemoteFrame=off  SimulateUsing=Code generation
  Digital Clock : DigitalClock  SampleTime=-1
  Divide : Product  Inputs=*/
  Max : MinMax  Function=max  Inputs=2
  Min : MinMax  Inputs=2
  Unit Delay : UnitDelay  SampleTime=-1  HasFrameUpgradeWarning=on
  Unit Delay1 : UnitDelay  InitialCondition=100  SampleTime=-1  HasFrameUpgradeWarning=on
  deg to % : MATLAB Function  TreatAsAtomicUnit=on
  kWH (need to redo after finding variant!!!!) : Constant  Value=80
  wires:
  CAN Pack64/1 -> CAN Transmit64/1
  Current Battery Temp/1 -> deg to %/1(battTempC)
  kWH (need to redo after finding variant!!!!)/1 -> CAN Pack64/2
  Divide/1 -> CAN Pack64/4
  SOC/1 -> CAN Pack64/3, Max/1, Min/1
  Max/1 -> Unit Delay/1, CAN Pack64/5
  Min/1 -> Unit Delay1/1, CAN Pack64/6
  Integrated SOC/1 -> Divide/1
  Digital Clock/1 -> Divide/2
  deg to %/1(battTempPct) -> CAN Pack64/1
  Unit Delay/1 -> Max/2
  Unit Delay1/1 -> Min/2

== system FYP/BMS Sum Charge ==
  Power1 : Inport
  Power2 : Inport  Port=2
  Trigger : TriggerPort  VariantControl=(inherit)
  CAN Pack106 : canmsglib/CAN Pack  CANdbFile=C:\Users\aaron\OneDrive - Loughborough University\Work\Part D\FYP\tesla sniffing\Model3CAN.dbc  MsgList=ID3D2TotalChargeDischarge  MsgName=ID3D2TotalChargeDischarge  MsgIDType=Standard (11-bit identifier)  MsgIdentifier=978  MsgLength=8  Remote=off  ApplyMinMax=off  BusOutput=on  SignalInfo={'TotalChargeKWh3D2','32','32','LE','unsigned','Standard','0','0.001','0','0','4294970';'TotalDischargeKWh3D2','0','32','LE','unsigned','Standard','0','0.001','0','0','4294970'}
      settings: LibrarySourceBlock=canlib/CAN Pack  DataFormat=CANdb specified signals
  CAN Transmit106 : raspberrypiCommlib/CAN Transmit  DeviceID=can0  SetupCAN=off  TypeofCAN=Real  InputDataType=CAN Msg  BlockingMode_=off  BlockTimeout_=1  OutputStatus=off  IdentifierType=Standard (11-bit identifier)  MessageId=100  MsgLength=8  RemoteFrame=off  SimulateUsing=Code generation
  Gain : Gain  Gain=1/60
  Gain1 : Gain  Gain=1/60
  wires:
  CAN Pack106/1 -> CAN Transmit106/1
  Power1/1 -> Gain/1
  Gain/1 -> CAN Pack106/1
  Gain1/1 -> CAN Pack106/2
  Power2/1 -> Gain1/1

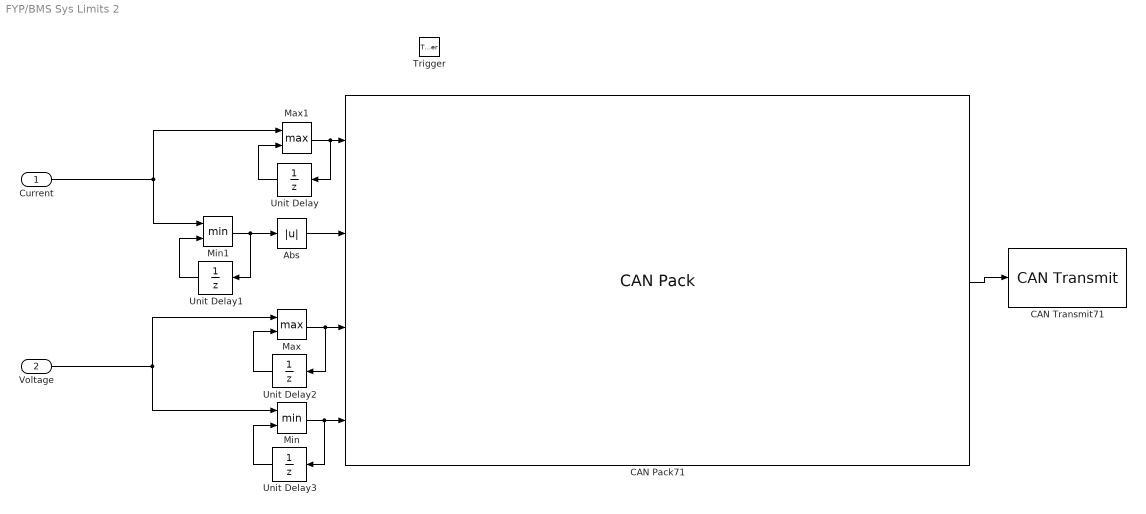
== system FYP/BMS Sys Limits 2 ==
  Current : Inport
  Voltage : Inport  Port=2
  Trigger : TriggerPort  VariantControl=(inherit)
  Abs : Abs  SaturateOnIntegerOverflow=off
  CAN Pack71 : canmsglib/CAN Pack  CANdbFile=C:\Users\aaron\OneDrive - Loughborough University\Work\Part D\FYP\tesla sniffing\Model3CAN.dbc  MsgList=ID2D2BMSVAlimits  MsgName=ID2D2BMSVAlimits  MsgIDType=Standard (11-bit identifier)  MsgIdentifier=722  MsgLength=8  Remote=off  ApplyMinMax=off  BusOutput=on  SignalInfo={'MaxChargeCurrent2D2','32','14','LE','unsigned','Standard','0','0.1','0','0','1638.2';'MaxDischargeCurrent2D2','48','14','LE','unsigned','Standard','0','0.128','0','0','2096.9';'MaxVoltage2D2','16','16','LE','unsigned','Standard','0','0.01','0','0','430';'MinVoltage2D2','0','16','LE','unsigned','Standard','0','0.01','0','0','430'}
      settings: LibrarySourceBlock=canlib/CAN Pack  DataFormat=CANdb specified signals
  CAN Transmit71 : raspberrypiCommlib/CAN Transmit  DeviceID=can0  SetupCAN=off  TypeofCAN=Real  InputDataType=CAN Msg  BlockingMode_=off  BlockTimeout_=1  OutputStatus=off  IdentifierType=Standard (11-bit identifier)  MessageId=100  MsgLength=8  RemoteFrame=off  SimulateUsing=Code generation
  Max : MinMax  Function=max  Inputs=2
  Max1 : MinMax  Function=max  Inputs=2
  Min : MinMax  Inputs=2
  Min1 : MinMax  Inputs=2
  Unit Delay : UnitDelay  SampleTime=-1  HasFrameUpgradeWarning=on
  Unit Delay1 : UnitDelay  InitialCondition=99999999  SampleTime=-1  HasFrameUpgradeWarning=on
  Unit Delay2 : UnitDelay  SampleTime=-1  HasFrameUpgradeWarning=on
  Unit Delay3 : UnitDelay  InitialCondition=999  SampleTime=-1  HasFrameUpgradeWarning=on
  wires:
  CAN Pack71/1 -> CAN Transmit71/1
  Min/1 -> CAN Pack71/4, Unit Delay3/1
  Max/1 -> CAN Pack71/3, Unit Delay2/1
  Max1/1 -> CAN Pack71/1, Unit Delay/1
  Min1/1 -> Abs/1, Unit Delay1/1
  Current/1 -> Min1/1, Max1/1
  Voltage/1 -> Min/1, Max/1
  Abs/1 -> CAN Pack71/2
  Unit Delay/1 -> Max1/2
  Unit Delay1/1 -> Min1/2
  Unit Delay2/1 -> Max/2
  Unit Delay3/1 -> Min/2

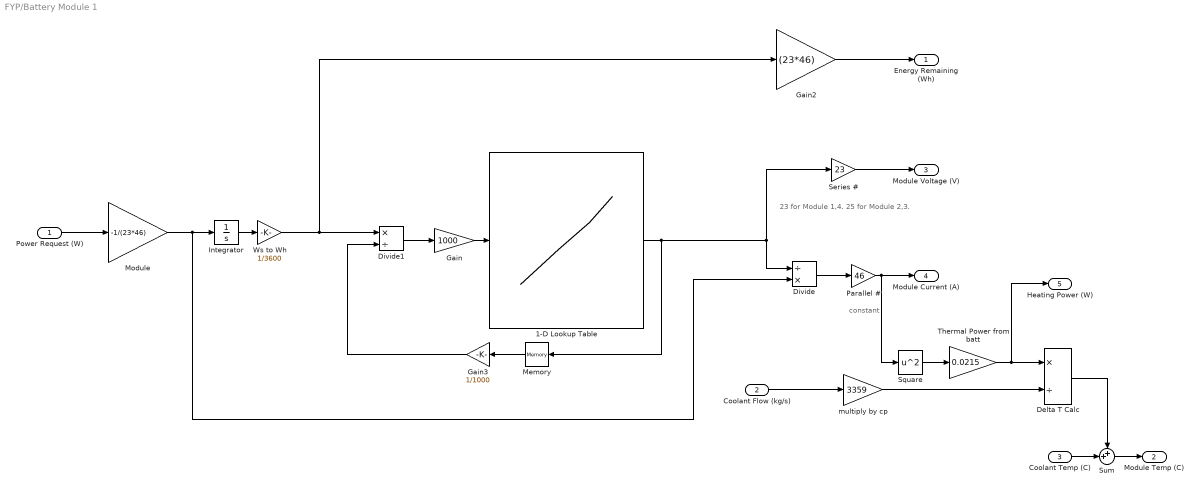
== system FYP/Battery Module 1 ==
  note: constant
  note: 23 for Module 1,4. 25 for Module 2,3.
  Power Request (W) : Inport
  Coolant Flow (kg/s) : Inport  Port=2
  Coolant Temp (C) : Inport  Port=3
  1-D Lookup Table : Lookup_n-D  NumberOfTableDimensions=1  BreakpointsForDimension1=|  Table=|  InternalRulePriority=Speed  RndMeth=Simplest
      BreakpointsForDimension1=|
      | [327.91963
      | 356.24194
      | 389.81097
      | 421.58966
      | 454.48731
      | 486.26599
      | 520.63596
      | 557.87992
      | 595.92482
      | 631.52398
      | 652.73854
      | 690.13124
      | 726.46639
      | 758.34729
      | 795.18499
      | 822.76755
      | 860.65393
      | 891.58806
      | 925.87788
      | 957.35139
      | 996.24173
      | 1029.9537
      | 1071.4861
      | 1113.3355
      | 1155.1849
      | 1197.0343
      | 1238.8837
      |  1280.733
      | 1322.5824
      | 1364.4318
      | 1406.2812
      | 1448.1306
      |   1489.98
      | 1531.8294
      | 1573.6788
      | 1615.5282
      | 1657.3776
      |  1699.227
      | 1741.0764
      | 1782.9257
      | 1824.7751
      | 1866.6245
      | 1908.4739
      | 1950.3233
      | 1992.1727
      | 2034.0221
      | 2075.8715
      | 2117.7209
      | 2174.7882
      | 2212.8331
      | 2254.6825
      | 2296.5319
      | 2338.3813
      | 2380.2307
      | 2422.0801
      | 2463.9295
      | 2505.7789
      | 2547.6283
      | 2589.4777
      |  2631.327
      | 2673.1764
      | 2715.0258
      | 2756.8752
      | 2798.7246
      |  2840.574
      | 2882.4234
      | 2924.2728
      | 2966.1222
      | 3007.9716
      |  3049.821
      | 3091.6704
      | 3133.5197
      | 3175.3691
      | 3217.2185
      | 3259.0679
      | 3300.9173
      | 3342.7667
      | 3384.6161
      | 3426.4655
      | 3468.3149
      | 3510.1643
      | 3552.0137
      | 3593.8631
      | 3635.7124
      | 3677.5618
      | 3719.4112
      | 3761.2606
      |   3803.11
      | 3844.9594
      | 3886.8088
      | 3928.6582
      | 3970.5076
      |  4012.357
      | 4054.2064
      | 4096.0558
      | 4137.9051
      | 4179.7545
      | 4221.6039
      | 4263.4533
      | 4305.3027
      | 4347.1521
      | 4389.0015
      | 4430.8509
      | 4472.7003
      | 4514.5497
      | 4556.3991
      | 4598.2485
      | 4640.0978
      | 4681.9472
      | 4704.0825
      | 4723.7966
      | 4748.3529
      |  4765.646
      | 4785.5464]
      Table=|
      | [2.7985
      | 2.8174
      | 2.8458
      | 2.8738
      | 2.8997
      | 2.9268
      | 2.9549
      | 2.9821
      |  3.009
      | 3.0311
      | 3.0525
      | 3.0727
      | 3.0956
      | 3.1205
      | 3.1365
      | 3.1586
      | 3.1795
      | 3.2002
      | 3.2177
      | 3.2408
      | 3.2608
      | 3.2799
      | 3.3019
      | 3.3209
      |  3.339
      | 3.3545
      | 3.3694
      | 3.3827
      | 3.3945
      | 3.4061
      | 3.4165
      | 3.4265
      |  3.436
      | 3.4452
      | 3.4545
      | 3.4628
      | 3.4712
      |  3.479
      | 3.4866
      | 3.4941
      | 3.5018
      | 3.5098
      | 3.5177
      | 3.5261
      | 3.5347
      | 3.5428
      | 3.5516
      |  3.558
      | 3.5778
      | 3.5818
      |  3.592
      | 3.6021
      | 3.6124
      | 3.6225
      | 3.6324
      | 3.6423
      | 3.6517
      |  3.661
      | 3.6705
      | 3.6797
      | 3.6889
      | 3.6981
      | 3.7063
      | 3.7141
      | 3.7223
      | 3.7297
      | 3.7373
      | 3.7442
      | 3.7511
      | 3.7579
      | 3.7643
      | 3.7711
      | 3.7777
      | 3.7847
      | 3.7916
      | 3.7991
      | 3.8065
      | 3.8143
      | 3.8224
      | 3.8311
      | 3.8405
      | 3.8501
      |   3.86
      | 3.8705
      | 3.8803
      | 3.8902
      |    3.9
      |  3.909
      | 3.9181
      | 3.9258
      | 3.9329
      | 3.9399
      | 3.9456
      | 3.9511
      | 3.9558
      | 3.9603
      | 3.9646
      | 3.9685
      | 3.9719
      |  3.975
      | 3.9783
      | 3.9817
      |  3.986
      | 3.9895
      | 3.9951
      | 4.0003
      | 4.0067
      | 4.0149
      | 4.0239
      | 4.0482
      | 4.0793
      | 4.1102
      | 4.1378
      | 4.1651]
  Delta T Calc : Product  Inputs=*/
  Divide : Product  Inputs=/*
  Divide1 : Product  Inputs=*/
  Gain : Gain  Gain=1000
  Gain2 : Gain  Gain=(23*46)
  Gain3 : Gain  Gain=1/1000
  Integrator : Integrator  InitialCondition=19.93*3600
  Memory : Memory  InitialCondition=4.1651
  "Module " : Gain  Gain=-1/(23*46)
  Parallel # : Gain  Gain=46
  Series # : Gain  Gain=23
  Square : Math  Operator=square
  Sum : Sum  Inputs=++|
  Thermal Power from batt : Gain  Gain=0.0215
  Ws to Wh : Gain  Gain=1/3600
  multiply by cp : Gain  Gain=3359
  Energy Remaining (Wh) : Outport
  Module Temp (C) : Outport  Port=2
  Module Voltage (V) : Outport  Port=3
  Module Current (A) : Outport  Port=4
  Heating Power (W) : Outport  Port=5
  wires:
  1-D Lookup Table/1 -> Memory/1, Divide/1, Series #/1
  Power Request (W)/1 -> "Module "/1
  Gain/1 -> 1-D Lookup Table/1
  Integrator/1 -> Ws to Wh/1
  Divide/1 -> Parallel #/1
  "Module "/1 -> Integrator/1, Divide/2
  Gain2/1 -> Energy Remaining (Wh)/1
  Series #/1 -> Module Voltage (V)/1
  Parallel #/1 -> Square/1, Module Current (A)/1
  Square/1 -> Thermal Power from batt/1
  Thermal Power from batt/1 -> Heating Power (W)/1, Delta T Calc/1
  multiply by cp/1 -> Delta T Calc/2
  Coolant Flow (kg/s)/1 -> multiply by cp/1
  Sum/1 -> Module Temp (C)/1
  Coolant Temp (C)/1 -> Sum/2
  Delta T Calc/1 -> Sum/1
  Memory/1 -> Gain3/1
  Divide1/1 -> Gain/1
  Gain3/1 -> Divide1/2
  Ws to Wh/1 -> Divide1/1, Gain2/1

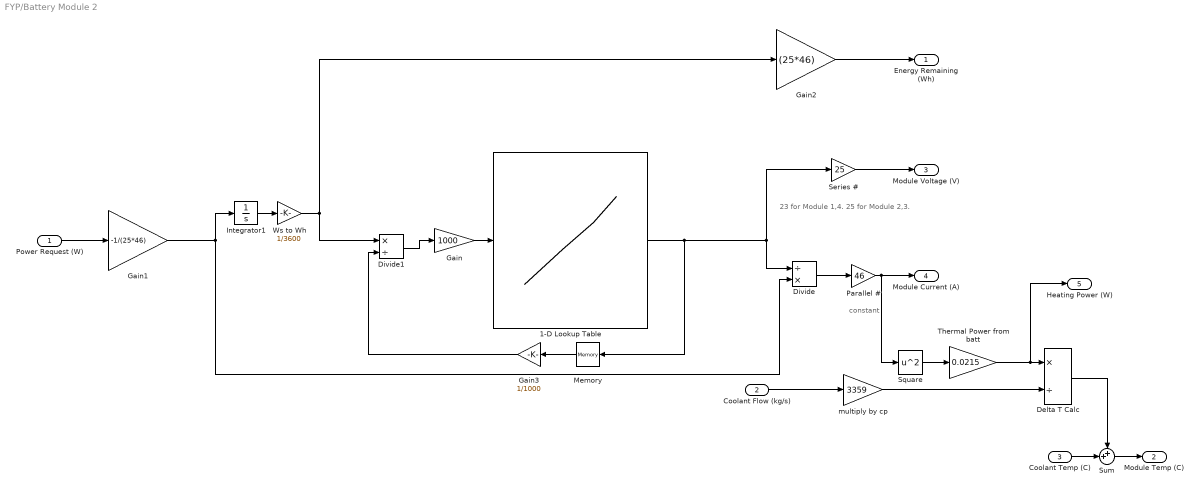
== system FYP/Battery Module 2 ==
  note: constant
  note: 23 for Module 1,4. 25 for Module 2,3.
  Power Request (W) : Inport
  Coolant Flow (kg/s) : Inport  Port=2
  Coolant Temp (C) : Inport  Port=3
  1-D Lookup Table : Lookup_n-D  NumberOfTableDimensions=1  BreakpointsForDimension1=|  Table=|  InternalRulePriority=Speed  RndMeth=Simplest
      BreakpointsForDimension1=|
      | [327.91963
      | 356.24194
      | 389.81097
      | 421.58966
      | 454.48731
      | 486.26599
      | 520.63596
      | 557.87992
      | 595.92482
      | 631.52398
      | 652.73854
      | 690.13124
      | 726.46639
      | 758.34729
      | 795.18499
      | 822.76755
      | 860.65393
      | 891.58806
      | 925.87788
      | 957.35139
      | 996.24173
      | 1029.9537
      | 1071.4861
      | 1113.3355
      | 1155.1849
      | 1197.0343
      | 1238.8837
      |  1280.733
      | 1322.5824
      | 1364.4318
      | 1406.2812
      | 1448.1306
      |   1489.98
      | 1531.8294
      | 1573.6788
      | 1615.5282
      | 1657.3776
      |  1699.227
      | 1741.0764
      | 1782.9257
      | 1824.7751
      | 1866.6245
      | 1908.4739
      | 1950.3233
      | 1992.1727
      | 2034.0221
      | 2075.8715
      | 2117.7209
      | 2174.7882
      | 2212.8331
      | 2254.6825
      | 2296.5319
      | 2338.3813
      | 2380.2307
      | 2422.0801
      | 2463.9295
      | 2505.7789
      | 2547.6283
      | 2589.4777
      |  2631.327
      | 2673.1764
      | 2715.0258
      | 2756.8752
      | 2798.7246
      |  2840.574
      | 2882.4234
      | 2924.2728
      | 2966.1222
      | 3007.9716
      |  3049.821
      | 3091.6704
      | 3133.5197
      | 3175.3691
      | 3217.2185
      | 3259.0679
      | 3300.9173
      | 3342.7667
      | 3384.6161
      | 3426.4655
      | 3468.3149
      | 3510.1643
      | 3552.0137
      | 3593.8631
      | 3635.7124
      | 3677.5618
      | 3719.4112
      | 3761.2606
      |   3803.11
      | 3844.9594
      | 3886.8088
      | 3928.6582
      | 3970.5076
      |  4012.357
      | 4054.2064
      | 4096.0558
      | 4137.9051
      | 4179.7545
      | 4221.6039
      | 4263.4533
      | 4305.3027
      | 4347.1521
      | 4389.0015
      | 4430.8509
      | 4472.7003
      | 4514.5497
      | 4556.3991
      | 4598.2485
      | 4640.0978
      | 4681.9472
      | 4704.0825
      | 4723.7966
      | 4748.3529
      |  4765.646
      | 4785.5464]
      Table=|
      | [2.7985
      | 2.8174
      | 2.8458
      | 2.8738
      | 2.8997
      | 2.9268
      | 2.9549
      | 2.9821
      |  3.009
      | 3.0311
      | 3.0525
      | 3.0727
      | 3.0956
      | 3.1205
      | 3.1365
      | 3.1586
      | 3.1795
      | 3.2002
      | 3.2177
      | 3.2408
      | 3.2608
      | 3.2799
      | 3.3019
      | 3.3209
      |  3.339
      | 3.3545
      | 3.3694
      | 3.3827
      | 3.3945
      | 3.4061
      | 3.4165
      | 3.4265
      |  3.436
      | 3.4452
      | 3.4545
      | 3.4628
      | 3.4712
      |  3.479
      | 3.4866
      | 3.4941
      | 3.5018
      | 3.5098
      | 3.5177
      | 3.5261
      | 3.5347
      | 3.5428
      | 3.5516
      |  3.558
      | 3.5778
      | 3.5818
      |  3.592
      | 3.6021
      | 3.6124
      | 3.6225
      | 3.6324
      | 3.6423
      | 3.6517
      |  3.661
      | 3.6705
      | 3.6797
      | 3.6889
      | 3.6981
      | 3.7063
      | 3.7141
      | 3.7223
      | 3.7297
      | 3.7373
      | 3.7442
      | 3.7511
      | 3.7579
      | 3.7643
      | 3.7711
      | 3.7777
      | 3.7847
      | 3.7916
      | 3.7991
      | 3.8065
      | 3.8143
      | 3.8224
      | 3.8311
      | 3.8405
      | 3.8501
      |   3.86
      | 3.8705
      | 3.8803
      | 3.8902
      |    3.9
      |  3.909
      | 3.9181
      | 3.9258
      | 3.9329
      | 3.9399
      | 3.9456
      | 3.9511
      | 3.9558
      | 3.9603
      | 3.9646
      | 3.9685
      | 3.9719
      |  3.975
      | 3.9783
      | 3.9817
      |  3.986
      | 3.9895
      | 3.9951
      | 4.0003
      | 4.0067
      | 4.0149
      | 4.0239
      | 4.0482
      | 4.0793
      | 4.1102
      | 4.1378
      | 4.1651]
  Delta T Calc : Product  Inputs=*/
  Divide : Product  Inputs=/*
  Divide1 : Product  Inputs=*/
  Gain : Gain  Gain=1000
  Gain1 : Gain  Gain=-1/(25*46)
  Gain2 : Gain  Gain=(25*46)
  Gain3 : Gain  Gain=1/1000
  Integrator1 : Integrator  InitialCondition=19.93*3600
  Memory : Memory  InitialCondition=4.1651
  Parallel # : Gain  Gain=46
  Series # : Gain  Gain=25
  Square : Math  Operator=square
  Sum : Sum  Inputs=++|
  Thermal Power from batt : Gain  Gain=0.0215
  Ws to Wh : Gain  Gain=1/3600
  multiply by cp : Gain  Gain=3359
  Energy Remaining (Wh) : Outport
  Module Temp (C) : Outport  Port=2
  Module Voltage (V) : Outport  Port=3
  Module Current (A) : Outport  Port=4
  Heating Power (W) : Outport  Port=5
  wires:
  1-D Lookup Table/1 -> Memory/1, Divide/1, Series #/1
  Power Request (W)/1 -> Gain1/1
  Gain/1 -> 1-D Lookup Table/1
  Ws to Wh/1 -> Divide1/1, Gain2/1
  Divide/1 -> Parallel #/1
  Gain1/1 -> Divide/2, Integrator1/1
  Gain2/1 -> Energy Remaining (Wh)/1
  Series #/1 -> Module Voltage (V)/1
  Parallel #/1 -> Square/1, Module Current (A)/1
  Square/1 -> Thermal Power from batt/1
  multiply by cp/1 -> Delta T Calc/2
  Coolant Flow (kg/s)/1 -> multiply by cp/1
  Sum/1 -> Module Temp (C)/1
  Coolant Temp (C)/1 -> Sum/2
  Delta T Calc/1 -> Sum/1
  Thermal Power from batt/1 -> Heating Power (W)/1, Delta T Calc/1
  Memory/1 -> Gain3/1
  Divide1/1 -> Gain/1
  Gain3/1 -> Divide1/2
  Integrator1/1 -> Ws to Wh/1
